simulink model "ortese_idb_pid_simulink_linear"  (R2024b)
settings: Solver=ode1  StartTime=0.0  StopTime=t_end  FixedStep=Ts  RelTol=1e-3
values from neighbouring files (symbols this model uses):
  A_mat = [0,                          1 ... (first row only)    [rodar_simulink_linear_test.m]
  B_mat = [0; 1/D11]    [rodar_simulink_linear_test.m]
  b_visc = 0.5    [rodar_simulink_linear_test.m]
  C_mat = [1, 0]    [rodar_simulink_linear_test.m]
  D11 = m*l_link^2/3 + m*r^2/4    (= 0.215833333333)    [rodar_simulink_linear_test.m]
  D_mat = 0    [rodar_simulink_linear_test.m]
  Kd = D11*wn_d*(2*zeta_d + alpha_d) - b_visc    (= 16.076)    [rodar_simulink_linear_test.m]
  Ki = D11*alpha_d*wn_d^3    (= 884.053333333)    [rodar_simulink_linear_test.m]
  Kp = D11*wn_d^2*(1 + 2*zeta_d*alpha_d)    (= 190.624)    [rodar_simulink_linear_test.m]
  mgd = m*g*d    (= 7.848)    [rodar_simulink_linear_test.m]
  tau_eq_lin = mgd*cos(theta0_lin)    [rodar_simulink_linear_test.m]
  tau_max = 200    [rodar_simulink_linear_test.m]
  theta0_lin = mean(ref)    [rodar_simulink_linear_test.m]
  Ts = 1e-3    (= 0.001)    [rodar_simulink_linear_test.m]
  x_init_lin = [ref(1) - theta0_lin ... (first row only)    [rodar_simulink_linear_test.m]
libraries: slpidlib x1
settings Model: Creator=anton  LastModifiedBy=anton

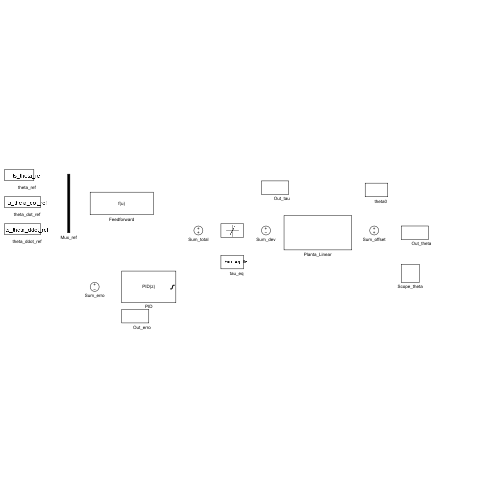
[thumbnail: Simulink's stored preview of the top-level diagram]
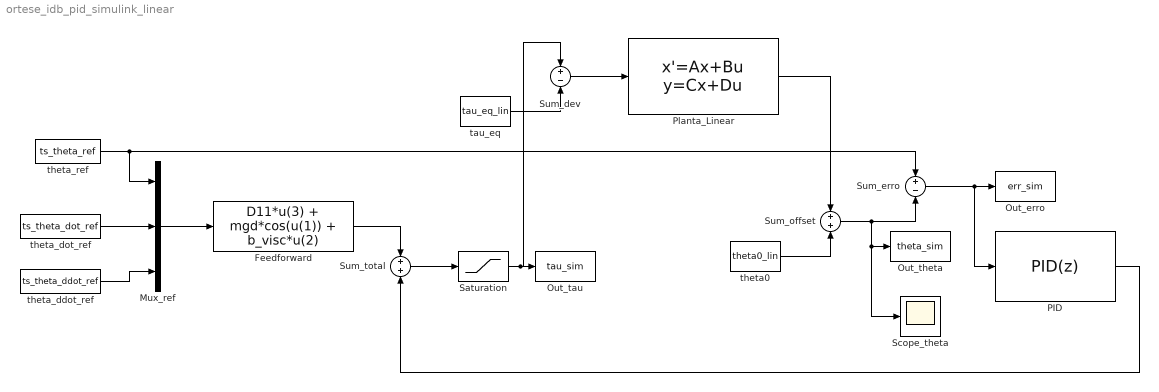
== system ortese_idb_pid_simulink_linear ==
  Feedforward : Fcn  Expr=D11*u(3) + mgd*cos(u(1)) + b_visc*u(2)
  Mux_ref : Mux  Inputs=3
  Out_erro : ToWorkspace  VariableName=err_sim  SaveFormat=Timeseries  SampleTime=-1
  Out_tau : ToWorkspace  VariableName=tau_sim  SaveFormat=Timeseries  SampleTime=-1
  Out_theta : ToWorkspace  VariableName=theta_sim  SaveFormat=Timeseries  SampleTime=-1
  PID : slpidlib/PID Controller  Controller=PID  Form=Parallel  TimeDomain=Discrete-time  UseExternalTs=off  SampleTime=Ts  IntegratorMethod=Forward Euler  FilterMethod=Backward Euler  ControllerParametersSource=internal  P=Kp  I=Ki  UseKiTs=off  D=Kd  UseExternalDerivativeSource=off  N=100  UseFilter=off  TunerSelectOption=Transfer Function Based (PID Tuner App)  InitialConditionSource=internal  InitialConditionForIntegrator=0  InitialConditionForFilter=0  DifferentiatorICPrevScaledInput=0  ExternalReset=none  TrackingMode=off  Kt=1  LimitOutput=on  SatLimitsSource=internal  UpperSaturationLimit=tau_max  LowerSaturationLimit=-tau_max  LinearizeAsGain=on  AntiWindupMode=back-calculation  Kb=1  LimitIntegrator=off  UpperIntegratorSaturationLimit=inf  LowerIntegratorSaturationLimit=-inf  POutMin=[]  POutMax=[]  IOutMin=[]  IOutMax=[]  DOutMin=[]  DOutMax=[]  NOutMin=[]  NOutMax=[]  SumOutMin=[]  SumOutMax=[]  SaturationOutMin=[]  SaturationOutMax=[]  PParamMin=[]  PParamMax=[]  IParamMin=[]  IParamMax=[]  DParamMin=[]  DParamMax=[]  NParamMin=[]  NParamMax=[]  KbParamMin=[]  KbParamMax=[]  KtParamMin=[]  KtParamMax=[]  KbOutMin=[]  KbOutMax=[]  KtOutMin=[]  KtOutMax=[]  IntegratorOutMin=[]  IntegratorOutMax=[]  FilterOutMin=[]  FilterOutMax=[]  SumI1OutMin=[]  SumI1OutMax=[]  SumI2OutMin=[]  SumI2OutMax=[]  SumI3OutMin=[]  SumI3OutMax=[]  SumI4OutMin=[]  SumI4OutMax=[]  SumDOutMin=[]  SumDOutMax=[]  DifferentiatorOutMin=[]  DifferentiatorOutMax=[]  FilterDiffOutCoefMin=[]  FilterDiffOutCoefMax=[]  ReciprocalOutMin=[]  ReciprocalOutMax=[]  SumDenOutMin=[]  SumDenOutMax=[]  SumNumOutMin=[]  SumNumOutMax=[]  DivideOutMin=[]  DivideOutMax=[]  UdiffTsProdOutMin=[]  UdiffTsProdOutMax=[]  NTsProdOutMin=[]  NTsProdOutMax=[]  UintegralTsProdOutMin=[]  UintegralTsProdOutMax=[]  UngainTsProdOutMin=[]  UngainTsProdOutMax=[]  ClampingZeroOutDataTypeStr=Inherit: Inherit via back propagation  ClampingZeroOutMin=[]  ClampingZeroOutMax=[]  FilterDenConstantOutDataTypeStr=Inherit: Inherit via back propagation  FilterDenConstantOutMin=[]  FilterDenConstantOutMax=[]  PCopyOutDataTypeStr=Inherit: Inherit via back propagation  PCopyOutMin=[]  PCopyOutMax=[]  NCopyOutDataTypeStr=Inherit: Inherit via back propagation  NCopyOutMin=[]  NCopyOutMax=[]  IntegratorContinuousStateAttributes=''  IntegratorStateMustResolveToSignalObject=off  IntegratorRTWStateStorageClass=Auto  FilterContinuousStateAttributes=''  FilterStateMustResolveToSignalObject=off  FilterRTWStateStorageClass=Auto  ParallelPVariant=InternalParameters  IdealPVariant=Disabled  IVariant=InternalParameters  DVariant=InternalParameters  IntegratorVariant=Discrete  SatVariant=Enabled  AWVariant=BackCalculation  PCopyVariant=Disabled  TRVariant=Disabled  FdbkBlocksVariant=Forward  IdealPFdbkVariant=Disabled  SatFdbkVariant=Disabled  DerivativeFilterVariant=Differentiator  NVariant=Passthrough  NCopyVariant=Disabled_SignalSpec  FilterICVariant=InternalICsDifferentiator  IntegratorICVariant=InternalICs  ExternalResetVariant=Disabled  TRSumVariant=Passthrough  SumFdbkVariant=Disabled  SumVariant=Sum_PID  TsampFilterVariant=InternalTs  TsampNgainVariant=Passthrough  TsampIntegralVariant=Disabled_SignalSpec  ExternalSaturationOutDataTypeStr=Inherit: Same as second input  DerivativeSourceVariant=ErrorSignal  PreIntVariant=InternalPreInt
  Planta_Linear : StateSpace  A=A_mat  B=B_mat  C=C_mat  D=D_mat  InitialCondition=x_init_lin
  Saturation : Saturate  UpperLimit=tau_max  LowerLimit=-tau_max
  Scope_theta : Scope
  Sum_dev : Sum  Inputs=+-
  Sum_erro : Sum  Inputs=+-
  Sum_offset : Sum
  Sum_total : Sum
  tau_eq : Constant  Value=tau_eq_lin
  theta0 : Constant  Value=theta0_lin
  theta_ddot_ref : FromWorkspace  VariableName=ts_theta_ddot_ref
  theta_dot_ref : FromWorkspace  VariableName=ts_theta_dot_ref
  theta_ref : FromWorkspace  VariableName=ts_theta_ref
  wires:
  theta_ref/1 -> Sum_erro/1, Mux_ref/1
  theta_dot_ref/1 -> Mux_ref/2
  theta_ddot_ref/1 -> Mux_ref/3
  Mux_ref/1 -> Feedforward/1
  Sum_total/1 -> Saturation/1
  Feedforward/1 -> Sum_total/1
  tau_eq/1 -> Sum_dev/2
  Saturation/1 -> Sum_dev/1, Out_tau/1
  Sum_dev/1 -> Planta_Linear/1
  Planta_Linear/1 -> Sum_offset/1
  theta0/1 -> Sum_offset/2
  Sum_offset/1 -> Out_theta/1, Scope_theta/1, Sum_erro/2
  Sum_erro/1 -> PID/1, Out_erro/1
  PID/1 -> Sum_total/2
